simulink model "Assignment3_troubleshoot"  (R2024b)
settings: Solver=VariableStepAuto  StartTime=0.0  StopTime=0.35  MaxStep=1e-5  RelTol=1e-3
values from neighbouring files (symbols this model uses):
  C_sm = 5e-3    (= 0.005)    [assignment3.m]    (also in matlab.mat)
  Larm = 3e-3    (= 0.003)    [assignment3.m]    (also in matlab.mat)
libraries: spsIGBTDiodeLib x48, spsSeriesRLCBranchLib x30, spsVoltageMeasurementLib x28, spsTriangleGeneratorLib x24, spsCurrentMeasurementLib x9, slpidlib x5, spsabctodq0Lib x3, eeSinGeneratorThreePhase x2, spsdq0toabcLib x2, spsDCVoltageSourceLib x1, spsGroundLib x1, eePowerMeasurement x1
(part 2 of 2)

== system Assignment3_troubleshoot/Subsystem19 ==
  g : Inport
  IGBT/Diode : spsIGBTDiodeLib/IGBT//Diode  Ron=1e-3  Rs=1e5  Cs=inf  Measurements=off
  IGBT/Diode1 : spsIGBTDiodeLib/IGBT//Diode  Ron=1e-3  Rs=1e5  Cs=inf  Measurements=off
  NOT : Logic  Operator=NOT  IconShape=distinctive  AllPortsSameDT=off  OutDataTypeStr=boolean
  Series RLC Branch : spsSeriesRLCBranchLib/Series RLC Branch  LConnTagsString=__new0  RConnTagsString=__new0  BranchType=C  Resistance=1  Inductance=1e-3  SetiL0=off  InitialCurrent=0  Capacitance=C_sm  Setx0=on  InitialVoltage=V_sm  Measurements=None
  Voltage Measurement : spsVoltageMeasurementLib/Voltage Measurement  PhasorSimulation=off  OutputType=Complex  PSBequivalent=0
  1 : PMIOPort  Side=Right
  2 : PMIOPort  Port=2  Side=Right
  tag scope: Vblow_sm4=global
  wires:
  NOT/1 -> IGBT/Diode1/1
  g/1 -> IGBT/Diode/1, NOT/1
  Voltage Measurement/1 -> [Vblow_sm4]
  connections:
  IGBT/Diode/RConn1 -- 1/RConn1 -- IGBT/Diode1/LConn1
  Series RLC Branch/LConn1 -- IGBT/Diode/LConn1 -- Voltage Measurement/LConn1
  Series RLC Branch/RConn1 -- 2/RConn1 -- IGBT/Diode1/RConn1 -- Voltage Measurement/LConn2

== system Assignment3_troubleshoot/Subsystem2 ==
  g : Inport
  IGBT/Diode : spsIGBTDiodeLib/IGBT//Diode  Ron=1e-3  Rs=1e5  Cs=inf  Measurements=off
  IGBT/Diode1 : spsIGBTDiodeLib/IGBT//Diode  Ron=1e-3  Rs=1e5  Cs=inf  Measurements=off
  NOT : Logic  Operator=NOT  IconShape=distinctive  AllPortsSameDT=off  OutDataTypeStr=boolean
  Series RLC Branch : spsSeriesRLCBranchLib/Series RLC Branch  LConnTagsString=__new0  RConnTagsString=__new0  BranchType=C  Resistance=1  Inductance=1e-3  SetiL0=off  InitialCurrent=0  Capacitance=C_sm  Setx0=on  InitialVoltage=V_sm  Measurements=None
  Voltage Measurement : spsVoltageMeasurementLib/Voltage Measurement  PhasorSimulation=off  OutputType=Complex  PSBequivalent=0
  1 : PMIOPort  Side=Right
  2 : PMIOPort  Port=2  Side=Right
  tag scope: Vaup_sm3=global
  wires:
  NOT/1 -> IGBT/Diode1/1
  g/1 -> IGBT/Diode/1, NOT/1
  Voltage Measurement/1 -> [Vaup_sm3]
  connections:
  IGBT/Diode/RConn1 -- 1/RConn1 -- IGBT/Diode1/LConn1
  Series RLC Branch/LConn1 -- IGBT/Diode/LConn1 -- Voltage Measurement/LConn1
  Series RLC Branch/RConn1 -- 2/RConn1 -- IGBT/Diode1/RConn1 -- Voltage Measurement/LConn2

== system Assignment3_troubleshoot/Subsystem20 ==
  g : Inport
  IGBT/Diode : spsIGBTDiodeLib/IGBT//Diode  Ron=1e-3  Rs=1e5  Cs=inf  Measurements=off
  IGBT/Diode1 : spsIGBTDiodeLib/IGBT//Diode  Ron=1e-3  Rs=1e5  Cs=inf  Measurements=off
  NOT : Logic  Operator=NOT  IconShape=distinctive  AllPortsSameDT=off  OutDataTypeStr=boolean
  Series RLC Branch : spsSeriesRLCBranchLib/Series RLC Branch  LConnTagsString=__new0  RConnTagsString=__new0  BranchType=C  Resistance=1  Inductance=1e-3  SetiL0=off  InitialCurrent=0  Capacitance=C_sm  Setx0=on  InitialVoltage=V_sm  Measurements=None
  Voltage Measurement : spsVoltageMeasurementLib/Voltage Measurement  PhasorSimulation=off  OutputType=Complex  PSBequivalent=0
  1 : PMIOPort  Side=Right
  2 : PMIOPort  Port=2  Side=Right
  tag scope: Vclow_sm1=global
  wires:
  NOT/1 -> IGBT/Diode1/1
  g/1 -> IGBT/Diode/1, NOT/1
  Voltage Measurement/1 -> [Vclow_sm1]
  connections:
  IGBT/Diode/RConn1 -- 1/RConn1 -- IGBT/Diode1/LConn1
  Series RLC Branch/LConn1 -- IGBT/Diode/LConn1 -- Voltage Measurement/LConn1
  Series RLC Branch/RConn1 -- 2/RConn1 -- IGBT/Diode1/RConn1 -- Voltage Measurement/LConn2

== system Assignment3_troubleshoot/Subsystem21 ==
  g : Inport
  IGBT/Diode : spsIGBTDiodeLib/IGBT//Diode  Ron=1e-3  Rs=1e5  Cs=inf  Measurements=off
  IGBT/Diode1 : spsIGBTDiodeLib/IGBT//Diode  Ron=1e-3  Rs=1e5  Cs=inf  Measurements=off
  NOT : Logic  Operator=NOT  IconShape=distinctive  AllPortsSameDT=off  OutDataTypeStr=boolean
  Series RLC Branch : spsSeriesRLCBranchLib/Series RLC Branch  LConnTagsString=__new0  RConnTagsString=__new0  BranchType=C  Resistance=1  Inductance=1e-3  SetiL0=off  InitialCurrent=0  Capacitance=C_sm  Setx0=on  InitialVoltage=V_sm  Measurements=None
  Voltage Measurement : spsVoltageMeasurementLib/Voltage Measurement  PhasorSimulation=off  OutputType=Complex  PSBequivalent=0
  1 : PMIOPort  Side=Right
  2 : PMIOPort  Port=2  Side=Right
  tag scope: Vclow_sm2=global
  wires:
  NOT/1 -> IGBT/Diode1/1
  g/1 -> IGBT/Diode/1, NOT/1
  Voltage Measurement/1 -> [Vclow_sm2]
  connections:
  IGBT/Diode/RConn1 -- 1/RConn1 -- IGBT/Diode1/LConn1
  Series RLC Branch/LConn1 -- IGBT/Diode/LConn1 -- Voltage Measurement/LConn1
  Series RLC Branch/RConn1 -- 2/RConn1 -- IGBT/Diode1/RConn1 -- Voltage Measurement/LConn2

== system Assignment3_troubleshoot/Subsystem22 ==
  g : Inport
  IGBT/Diode : spsIGBTDiodeLib/IGBT//Diode  Ron=1e-3  Rs=1e5  Cs=inf  Measurements=off
  IGBT/Diode1 : spsIGBTDiodeLib/IGBT//Diode  Ron=1e-3  Rs=1e5  Cs=inf  Measurements=off
  NOT : Logic  Operator=NOT  IconShape=distinctive  AllPortsSameDT=off  OutDataTypeStr=boolean
  Series RLC Branch : spsSeriesRLCBranchLib/Series RLC Branch  LConnTagsString=__new0  RConnTagsString=__new0  BranchType=C  Resistance=1  Inductance=1e-3  SetiL0=off  InitialCurrent=0  Capacitance=C_sm  Setx0=on  InitialVoltage=V_sm  Measurements=None
  Voltage Measurement : spsVoltageMeasurementLib/Voltage Measurement  PhasorSimulation=off  OutputType=Complex  PSBequivalent=0
  1 : PMIOPort  Side=Right
  2 : PMIOPort  Port=2  Side=Right
  tag scope: Vclow_sm3=global
  wires:
  NOT/1 -> IGBT/Diode1/1
  g/1 -> IGBT/Diode/1, NOT/1
  Voltage Measurement/1 -> [Vclow_sm3]
  connections:
  IGBT/Diode/RConn1 -- 1/RConn1 -- IGBT/Diode1/LConn1
  Series RLC Branch/LConn1 -- IGBT/Diode/LConn1 -- Voltage Measurement/LConn1
  Series RLC Branch/RConn1 -- 2/RConn1 -- IGBT/Diode1/RConn1 -- Voltage Measurement/LConn2

== system Assignment3_troubleshoot/Subsystem23 ==
  g : Inport
  IGBT/Diode : spsIGBTDiodeLib/IGBT//Diode  Ron=1e-3  Rs=1e5  Cs=inf  Measurements=off
  IGBT/Diode1 : spsIGBTDiodeLib/IGBT//Diode  Ron=1e-3  Rs=1e5  Cs=inf  Measurements=off
  NOT : Logic  Operator=NOT  IconShape=distinctive  AllPortsSameDT=off  OutDataTypeStr=boolean
  Series RLC Branch : spsSeriesRLCBranchLib/Series RLC Branch  LConnTagsString=__new0  RConnTagsString=__new0  BranchType=C  Resistance=1  Inductance=1e-3  SetiL0=off  InitialCurrent=0  Capacitance=C_sm  Setx0=on  InitialVoltage=V_sm  Measurements=None
  Voltage Measurement : spsVoltageMeasurementLib/Voltage Measurement  PhasorSimulation=off  OutputType=Complex  PSBequivalent=0
  1 : PMIOPort  Side=Right
  2 : PMIOPort  Port=2  Side=Right
  tag scope: Vclow_sm4=global
  wires:
  NOT/1 -> IGBT/Diode1/1
  g/1 -> IGBT/Diode/1, NOT/1
  Voltage Measurement/1 -> [Vclow_sm4]
  connections:
  IGBT/Diode/RConn1 -- 1/RConn1 -- IGBT/Diode1/LConn1
  Series RLC Branch/LConn1 -- IGBT/Diode/LConn1 -- Voltage Measurement/LConn1
  Series RLC Branch/RConn1 -- 2/RConn1 -- IGBT/Diode1/RConn1 -- Voltage Measurement/LConn2

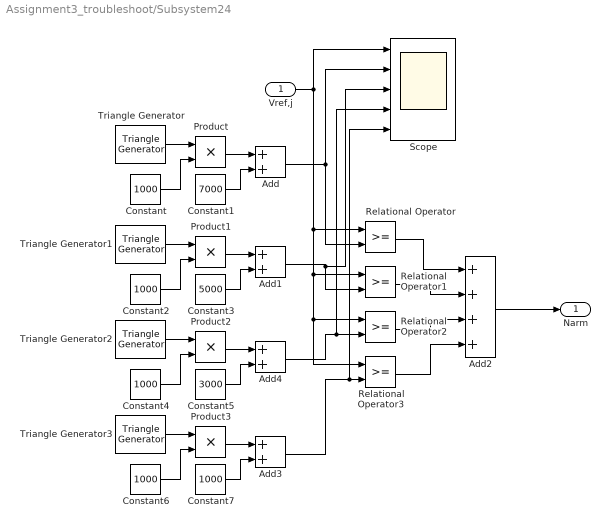
== system Assignment3_troubleshoot/Subsystem24 ==
  Vref,j : Inport
  Add{,1,3..4} (4 alike) : Sum
  Add2 : Sum  Inputs=++++
  Constant{,2,4,6..7} (5 alike) : Constant  Value=1000
  Constant1 : Constant  Value=7000
  Constant3 : Constant  Value=5000
  Constant5 : Constant  Value=3000
  Product{,1..3} (4 alike) : Product
  Relational Operator{,1..3} (4 alike) : RelationalOperator  OutDataTypeStr=boolean  RndMeth=Simplest  InputSameDT=off
  Scope : Scope  NumInputPorts=5
  Triangle Generator{,1..3} (4 alike) : spsTriangleGeneratorLib/Triangle Generator  Freq=1650  Phase=0  Ts=0
  Narm : Outport
  wires:
  Add/1 -> Relational Operator/2, Scope/2
  Product1/1 -> Add1/1
  Constant2/1 -> Product1/2
  Constant6/1 -> Product3/2
  Constant4/1 -> Product2/2
  Triangle Generator1/1 -> Product1/1
  Constant3/1 -> Add1/2
  Product3/1 -> Add3/1
  Add3/1 -> Scope/5, Relational Operator3/2
  Constant/1 -> Product/2
  Triangle Generator/1 -> Product/1
  Add1/1 -> Scope/3, Relational Operator1/2
  Add4/1 -> Scope/4, Relational Operator2/2
  Triangle Generator2/1 -> Product2/1
  Constant5/1 -> Add4/2
  Triangle Generator3/1 -> Product3/1
  Product/1 -> Add/1
  Add2/1 -> Narm/1
  Relational Operator/1 -> Add2/1
  Relational Operator3/1 -> Add2/4
  Constant1/1 -> Add/2
  Relational Operator2/1 -> Add2/3
  Vref,j/1 -> Relational Operator3/1, Relational Operator2/1, Relational Operator1/1, Relational Operator/1, Scope/1
  Constant7/1 -> Add3/2
  Relational Operator1/1 -> Add2/2
  Product2/1 -> Add4/1

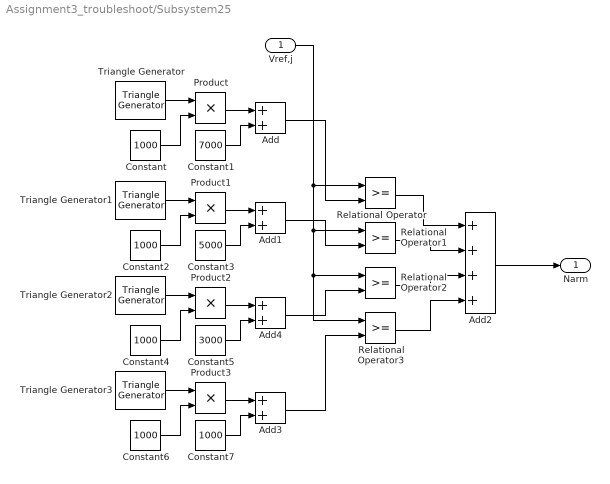
== system Assignment3_troubleshoot/Subsystem25 ==
  Vref,j : Inport
  Add{,1,3..4} (4 alike) : Sum
  Add2 : Sum  Inputs=++++
  Constant{,2,4,6..7} (5 alike) : Constant  Value=1000
  Constant1 : Constant  Value=7000
  Constant3 : Constant  Value=5000
  Constant5 : Constant  Value=3000
  Product{,1..3} (4 alike) : Product
  Relational Operator{,1..3} (4 alike) : RelationalOperator  OutDataTypeStr=boolean  RndMeth=Simplest  InputSameDT=off
  Triangle Generator{,1..3} (4 alike) : spsTriangleGeneratorLib/Triangle Generator  Freq=1650  Phase=0  Ts=0
  Narm : Outport
  wires:
  Add/1 -> Relational Operator/2
  Product1/1 -> Add1/1
  Constant2/1 -> Product1/2
  Constant6/1 -> Product3/2
  Constant4/1 -> Product2/2
  Triangle Generator1/1 -> Product1/1
  Constant3/1 -> Add1/2
  Product3/1 -> Add3/1
  Add3/1 -> Relational Operator3/2
  Constant/1 -> Product/2
  Triangle Generator/1 -> Product/1
  Add1/1 -> Relational Operator1/2
  Add4/1 -> Relational Operator2/2
  Triangle Generator2/1 -> Product2/1
  Constant5/1 -> Add4/2
  Triangle Generator3/1 -> Product3/1
  Product/1 -> Add/1
  Add2/1 -> Narm/1
  Relational Operator/1 -> Add2/1
  Relational Operator3/1 -> Add2/4
  Constant1/1 -> Add/2
  Relational Operator2/1 -> Add2/3
  Vref,j/1 -> Relational Operator3/1, Relational Operator2/1, Relational Operator1/1, Relational Operator/1
  Constant7/1 -> Add3/2
  Relational Operator1/1 -> Add2/2
  Product2/1 -> Add4/1

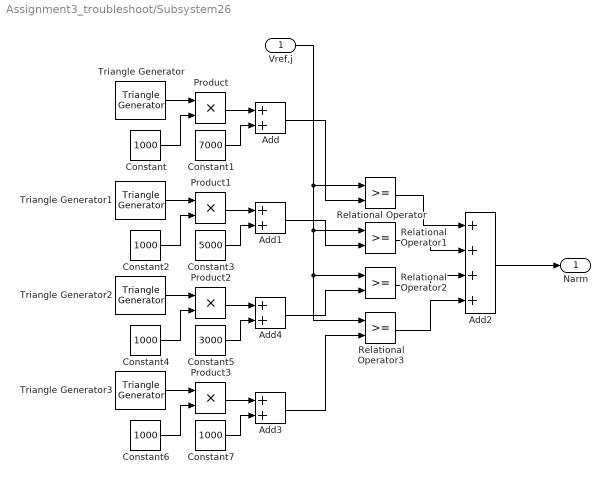
== system Assignment3_troubleshoot/Subsystem26 ==
  Vref,j : Inport
  Add{,1,3..4} (4 alike) : Sum
  Add2 : Sum  Inputs=++++
  Constant{,2,4,6..7} (5 alike) : Constant  Value=1000
  Constant1 : Constant  Value=7000
  Constant3 : Constant  Value=5000
  Constant5 : Constant  Value=3000
  Product{,1..3} (4 alike) : Product
  Relational Operator{,1..3} (4 alike) : RelationalOperator  OutDataTypeStr=boolean  RndMeth=Simplest  InputSameDT=off
  Triangle Generator{,1..3} (4 alike) : spsTriangleGeneratorLib/Triangle Generator  Freq=1650  Phase=0  Ts=0
  Narm : Outport
  wires:
  Add/1 -> Relational Operator/2
  Product1/1 -> Add1/1
  Constant2/1 -> Product1/2
  Constant6/1 -> Product3/2
  Constant4/1 -> Product2/2
  Triangle Generator1/1 -> Product1/1
  Constant3/1 -> Add1/2
  Product3/1 -> Add3/1
  Add3/1 -> Relational Operator3/2
  Constant/1 -> Product/2
  Triangle Generator/1 -> Product/1
  Add1/1 -> Relational Operator1/2
  Add4/1 -> Relational Operator2/2
  Triangle Generator2/1 -> Product2/1
  Constant5/1 -> Add4/2
  Triangle Generator3/1 -> Product3/1
  Product/1 -> Add/1
  Add2/1 -> Narm/1
  Relational Operator/1 -> Add2/1
  Relational Operator3/1 -> Add2/4
  Constant1/1 -> Add/2
  Relational Operator2/1 -> Add2/3
  Vref,j/1 -> Relational Operator3/1, Relational Operator2/1, Relational Operator1/1, Relational Operator/1
  Constant7/1 -> Add3/2
  Relational Operator1/1 -> Add2/2
  Product2/1 -> Add4/1

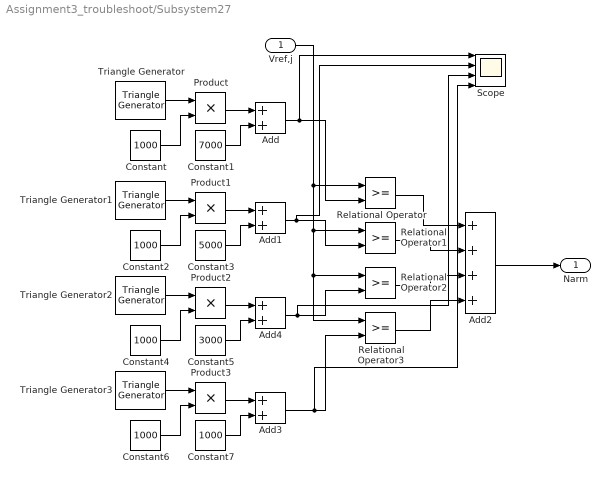
== system Assignment3_troubleshoot/Subsystem27 ==
  Vref,j : Inport
  Add{,1,3..4} (4 alike) : Sum
  Add2 : Sum  Inputs=++++
  Constant{,2,4,6..7} (5 alike) : Constant  Value=1000
  Constant1 : Constant  Value=7000
  Constant3 : Constant  Value=5000
  Constant5 : Constant  Value=3000
  Product{,1..3} (4 alike) : Product
  Relational Operator{,1..3} (4 alike) : RelationalOperator  OutDataTypeStr=boolean  RndMeth=Simplest  InputSameDT=off
  Scope : Scope  NumInputPorts=4
  Triangle Generator{,1..3} (4 alike) : spsTriangleGeneratorLib/Triangle Generator  Freq=1650  Phase=0  Ts=0
  Narm : Outport
  wires:
  Product1/1 -> Add1/1
  Constant2/1 -> Product1/2
  Constant6/1 -> Product3/2
  Constant4/1 -> Product2/2
  Triangle Generator1/1 -> Product1/1
  Constant3/1 -> Add1/2
  Product3/1 -> Add3/1
  Add3/1 -> Scope/4, Relational Operator3/2
  Constant/1 -> Product/2
  Triangle Generator/1 -> Product/1
  Add1/1 -> Scope/2, Relational Operator1/2
  Add4/1 -> Scope/3, Relational Operator2/2
  Triangle Generator2/1 -> Product2/1
  Constant5/1 -> Add4/2
  Triangle Generator3/1 -> Product3/1
  Product/1 -> Add/1
  Add2/1 -> Narm/1
  Relational Operator/1 -> Add2/1
  Relational Operator3/1 -> Add2/4
  Constant1/1 -> Add/2
  Relational Operator2/1 -> Add2/3
  Vref,j/1 -> Relational Operator3/1, Relational Operator2/1, Relational Operator1/1, Relational Operator/1
  Constant7/1 -> Add3/2
  Relational Operator1/1 -> Add2/2
  Product2/1 -> Add4/1
  Add/1 -> Scope/1, Relational Operator/2

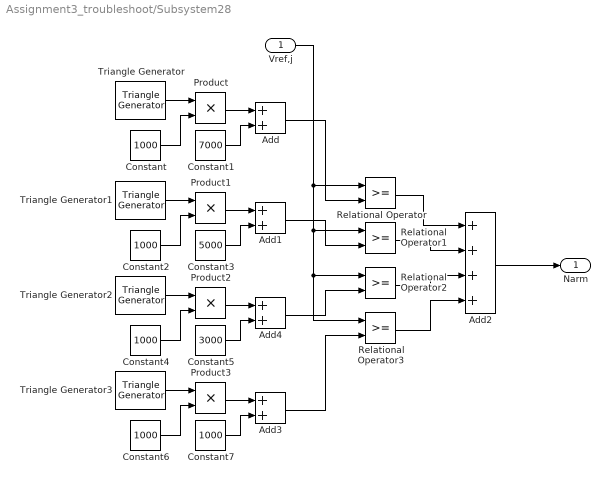
== system Assignment3_troubleshoot/Subsystem28 ==
  Vref,j : Inport
  Add{,1,3..4} (4 alike) : Sum
  Add2 : Sum  Inputs=++++
  Constant{,2,4,6..7} (5 alike) : Constant  Value=1000
  Constant1 : Constant  Value=7000
  Constant3 : Constant  Value=5000
  Constant5 : Constant  Value=3000
  Product{,1..3} (4 alike) : Product
  Relational Operator{,1..3} (4 alike) : RelationalOperator  OutDataTypeStr=boolean  RndMeth=Simplest  InputSameDT=off
  Triangle Generator{,1..3} (4 alike) : spsTriangleGeneratorLib/Triangle Generator  Freq=1650  Phase=0  Ts=0
  Narm : Outport
  wires:
  Add/1 -> Relational Operator/2
  Product1/1 -> Add1/1
  Constant2/1 -> Product1/2
  Constant6/1 -> Product3/2
  Constant4/1 -> Product2/2
  Triangle Generator1/1 -> Product1/1
  Constant3/1 -> Add1/2
  Product3/1 -> Add3/1
  Add3/1 -> Relational Operator3/2
  Constant/1 -> Product/2
  Triangle Generator/1 -> Product/1
  Add1/1 -> Relational Operator1/2
  Add4/1 -> Relational Operator2/2
  Triangle Generator2/1 -> Product2/1
  Constant5/1 -> Add4/2
  Triangle Generator3/1 -> Product3/1
  Product/1 -> Add/1
  Add2/1 -> Narm/1
  Relational Operator/1 -> Add2/1
  Relational Operator3/1 -> Add2/4
  Constant1/1 -> Add/2
  Relational Operator2/1 -> Add2/3
  Vref,j/1 -> Relational Operator3/1, Relational Operator2/1, Relational Operator1/1, Relational Operator/1
  Constant7/1 -> Add3/2
  Relational Operator1/1 -> Add2/2
  Product2/1 -> Add4/1

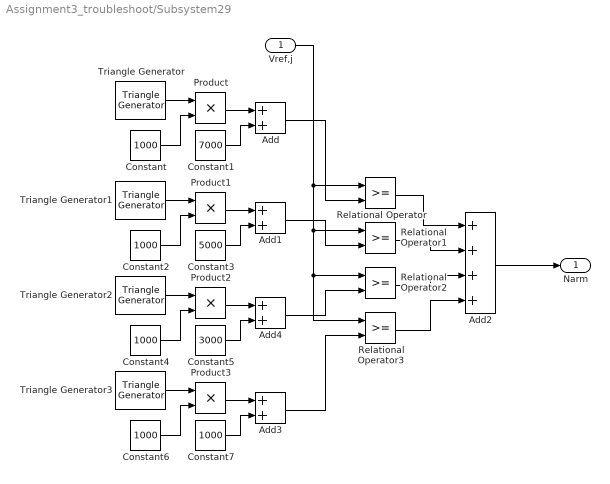
== system Assignment3_troubleshoot/Subsystem29 ==
  Vref,j : Inport
  Add{,1,3..4} (4 alike) : Sum
  Add2 : Sum  Inputs=++++
  Constant{,2,4,6..7} (5 alike) : Constant  Value=1000
  Constant1 : Constant  Value=7000
  Constant3 : Constant  Value=5000
  Constant5 : Constant  Value=3000
  Product{,1..3} (4 alike) : Product
  Relational Operator{,1..3} (4 alike) : RelationalOperator  OutDataTypeStr=boolean  RndMeth=Simplest  InputSameDT=off
  Triangle Generator{,1..3} (4 alike) : spsTriangleGeneratorLib/Triangle Generator  Freq=1650  Phase=0  Ts=0
  Narm : Outport
  wires:
  Add/1 -> Relational Operator/2
  Product1/1 -> Add1/1
  Constant2/1 -> Product1/2
  Constant6/1 -> Product3/2
  Constant4/1 -> Product2/2
  Triangle Generator1/1 -> Product1/1
  Constant3/1 -> Add1/2
  Product3/1 -> Add3/1
  Add3/1 -> Relational Operator3/2
  Constant/1 -> Product/2
  Triangle Generator/1 -> Product/1
  Add1/1 -> Relational Operator1/2
  Add4/1 -> Relational Operator2/2
  Triangle Generator2/1 -> Product2/1
  Constant5/1 -> Add4/2
  Triangle Generator3/1 -> Product3/1
  Product/1 -> Add/1
  Add2/1 -> Narm/1
  Relational Operator/1 -> Add2/1
  Relational Operator3/1 -> Add2/4
  Constant1/1 -> Add/2
  Relational Operator2/1 -> Add2/3
  Vref,j/1 -> Relational Operator3/1, Relational Operator2/1, Relational Operator1/1, Relational Operator/1
  Constant7/1 -> Add3/2
  Relational Operator1/1 -> Add2/2
  Product2/1 -> Add4/1

== system Assignment3_troubleshoot/Subsystem3 ==
  g : Inport
  IGBT/Diode : spsIGBTDiodeLib/IGBT//Diode  Ron=1e-3  Rs=1e5  Cs=inf  Measurements=off
  IGBT/Diode1 : spsIGBTDiodeLib/IGBT//Diode  Ron=1e-3  Rs=1e5  Cs=inf  Measurements=off
  NOT : Logic  Operator=NOT  IconShape=distinctive  AllPortsSameDT=off  OutDataTypeStr=boolean
  Series RLC Branch : spsSeriesRLCBranchLib/Series RLC Branch  LConnTagsString=__new0  RConnTagsString=__new0  BranchType=C  Resistance=1  Inductance=1e-3  SetiL0=off  InitialCurrent=0  Capacitance=C_sm  Setx0=on  InitialVoltage=V_sm  Measurements=None
  Voltage Measurement : spsVoltageMeasurementLib/Voltage Measurement  PhasorSimulation=off  OutputType=Complex  PSBequivalent=0
  1 : PMIOPort  Side=Right
  2 : PMIOPort  Port=2  Side=Right
  tag scope: Vaup_sm4=global
  wires:
  NOT/1 -> IGBT/Diode1/1
  g/1 -> IGBT/Diode/1, NOT/1
  Voltage Measurement/1 -> [Vaup_sm4]
  connections:
  IGBT/Diode/RConn1 -- 1/RConn1 -- IGBT/Diode1/LConn1
  Series RLC Branch/LConn1 -- IGBT/Diode/LConn1 -- Voltage Measurement/LConn1
  Series RLC Branch/RConn1 -- 2/RConn1 -- IGBT/Diode1/RConn1 -- Voltage Measurement/LConn2

== system Assignment3_troubleshoot/Subsystem4 ==
  g : Inport
  IGBT/Diode : spsIGBTDiodeLib/IGBT//Diode  Ron=1e-3  Rs=1e5  Cs=inf  Measurements=off
  IGBT/Diode1 : spsIGBTDiodeLib/IGBT//Diode  Ron=1e-3  Rs=1e5  Cs=inf  Measurements=off
  NOT : Logic  Operator=NOT  IconShape=distinctive  AllPortsSameDT=off  OutDataTypeStr=boolean
  Series RLC Branch : spsSeriesRLCBranchLib/Series RLC Branch  LConnTagsString=__new0  RConnTagsString=__new0  BranchType=C  Resistance=1  Inductance=1e-3  SetiL0=off  InitialCurrent=0  Capacitance=C_sm  Setx0=on  InitialVoltage=V_sm  Measurements=None
  Voltage Measurement : spsVoltageMeasurementLib/Voltage Measurement  PhasorSimulation=off  OutputType=Complex  PSBequivalent=0
  1 : PMIOPort  Side=Right
  2 : PMIOPort  Port=2  Side=Right
  tag scope: Valow_sm1=global
  wires:
  NOT/1 -> IGBT/Diode1/1
  g/1 -> IGBT/Diode/1, NOT/1
  Voltage Measurement/1 -> [Valow_sm1]
  connections:
  IGBT/Diode/RConn1 -- 1/RConn1 -- IGBT/Diode1/LConn1
  Series RLC Branch/LConn1 -- IGBT/Diode/LConn1 -- Voltage Measurement/LConn1
  Series RLC Branch/RConn1 -- 2/RConn1 -- IGBT/Diode1/RConn1 -- Voltage Measurement/LConn2

== system Assignment3_troubleshoot/Subsystem5 ==
  g : Inport
  IGBT/Diode : spsIGBTDiodeLib/IGBT//Diode  Ron=1e-3  Rs=1e5  Cs=inf  Measurements=off
  IGBT/Diode1 : spsIGBTDiodeLib/IGBT//Diode  Ron=1e-3  Rs=1e5  Cs=inf  Measurements=off
  NOT : Logic  Operator=NOT  IconShape=distinctive  AllPortsSameDT=off  OutDataTypeStr=boolean
  Series RLC Branch : spsSeriesRLCBranchLib/Series RLC Branch  LConnTagsString=__new0  RConnTagsString=__new0  BranchType=C  Resistance=1  Inductance=1e-3  SetiL0=off  InitialCurrent=0  Capacitance=C_sm  Setx0=on  InitialVoltage=V_sm  Measurements=None
  Voltage Measurement : spsVoltageMeasurementLib/Voltage Measurement  PhasorSimulation=off  OutputType=Complex  PSBequivalent=0
  1 : PMIOPort  Side=Right
  2 : PMIOPort  Port=2  Side=Right
  tag scope: Valow_sm2=global
  wires:
  NOT/1 -> IGBT/Diode1/1
  g/1 -> IGBT/Diode/1, NOT/1
  Voltage Measurement/1 -> [Valow_sm2]
  connections:
  IGBT/Diode/RConn1 -- 1/RConn1 -- IGBT/Diode1/LConn1
  Series RLC Branch/LConn1 -- IGBT/Diode/LConn1 -- Voltage Measurement/LConn1
  Series RLC Branch/RConn1 -- 2/RConn1 -- IGBT/Diode1/RConn1 -- Voltage Measurement/LConn2

== system Assignment3_troubleshoot/Subsystem6 ==
  g : Inport
  IGBT/Diode : spsIGBTDiodeLib/IGBT//Diode  Ron=1e-3  Rs=1e5  Cs=inf  Measurements=off
  IGBT/Diode1 : spsIGBTDiodeLib/IGBT//Diode  Ron=1e-3  Rs=1e5  Cs=inf  Measurements=off
  NOT : Logic  Operator=NOT  IconShape=distinctive  AllPortsSameDT=off  OutDataTypeStr=boolean
  Series RLC Branch : spsSeriesRLCBranchLib/Series RLC Branch  LConnTagsString=__new0  RConnTagsString=__new0  BranchType=C  Resistance=1  Inductance=1e-3  SetiL0=off  InitialCurrent=0  Capacitance=C_sm  Setx0=on  InitialVoltage=V_sm  Measurements=None
  Voltage Measurement : spsVoltageMeasurementLib/Voltage Measurement  PhasorSimulation=off  OutputType=Complex  PSBequivalent=0
  1 : PMIOPort  Side=Right
  2 : PMIOPort  Port=2  Side=Right
  tag scope: Valow_sm3=global
  wires:
  NOT/1 -> IGBT/Diode1/1
  g/1 -> IGBT/Diode/1, NOT/1
  Voltage Measurement/1 -> [Valow_sm3]
  connections:
  IGBT/Diode/RConn1 -- 1/RConn1 -- IGBT/Diode1/LConn1
  Series RLC Branch/LConn1 -- IGBT/Diode/LConn1 -- Voltage Measurement/LConn1
  Series RLC Branch/RConn1 -- 2/RConn1 -- IGBT/Diode1/RConn1 -- Voltage Measurement/LConn2

== system Assignment3_troubleshoot/Subsystem7 ==
  g : Inport
  IGBT/Diode : spsIGBTDiodeLib/IGBT//Diode  Ron=1e-3  Rs=1e5  Cs=inf  Measurements=off
  IGBT/Diode1 : spsIGBTDiodeLib/IGBT//Diode  Ron=1e-3  Rs=1e5  Cs=inf  Measurements=off
  NOT : Logic  Operator=NOT  IconShape=distinctive  AllPortsSameDT=off  OutDataTypeStr=boolean
  Series RLC Branch : spsSeriesRLCBranchLib/Series RLC Branch  LConnTagsString=__new0  RConnTagsString=__new0  BranchType=C  Resistance=1  Inductance=1e-3  SetiL0=off  InitialCurrent=0  Capacitance=C_sm  Setx0=on  InitialVoltage=V_sm  Measurements=None
  Voltage Measurement : spsVoltageMeasurementLib/Voltage Measurement  PhasorSimulation=off  OutputType=Complex  PSBequivalent=0
  1 : PMIOPort  Side=Right
  2 : PMIOPort  Port=2  Side=Right
  tag scope: Valow_sm4=global
  wires:
  NOT/1 -> IGBT/Diode1/1
  g/1 -> IGBT/Diode/1, NOT/1
  Voltage Measurement/1 -> [Valow_sm4]
  connections:
  IGBT/Diode/RConn1 -- 1/RConn1 -- IGBT/Diode1/LConn1
  Series RLC Branch/LConn1 -- IGBT/Diode/LConn1 -- Voltage Measurement/LConn1
  Series RLC Branch/RConn1 -- 2/RConn1 -- IGBT/Diode1/RConn1 -- Voltage Measurement/LConn2

== system Assignment3_troubleshoot/Subsystem8 ==
  g : Inport
  IGBT/Diode : spsIGBTDiodeLib/IGBT//Diode  Ron=1e-3  Rs=1e5  Cs=inf  Measurements=off
  IGBT/Diode1 : spsIGBTDiodeLib/IGBT//Diode  Ron=1e-3  Rs=1e5  Cs=inf  Measurements=off
  NOT : Logic  Operator=NOT  IconShape=distinctive  AllPortsSameDT=off  OutDataTypeStr=boolean
  Series RLC Branch : spsSeriesRLCBranchLib/Series RLC Branch  LConnTagsString=__new0  RConnTagsString=__new0  BranchType=C  Resistance=1  Inductance=1e-3  SetiL0=off  InitialCurrent=0  Capacitance=C_sm  Setx0=on  InitialVoltage=V_sm  Measurements=None
  Voltage Measurement : spsVoltageMeasurementLib/Voltage Measurement  PhasorSimulation=off  OutputType=Complex  PSBequivalent=0
  1 : PMIOPort  Side=Right
  2 : PMIOPort  Port=2  Side=Right
  tag scope: Vbup_sm1=global
  wires:
  NOT/1 -> IGBT/Diode1/1
  g/1 -> IGBT/Diode/1, NOT/1
  Voltage Measurement/1 -> [Vbup_sm1]
  connections:
  IGBT/Diode/RConn1 -- 1/RConn1 -- IGBT/Diode1/LConn1
  Series RLC Branch/LConn1 -- IGBT/Diode/LConn1 -- Voltage Measurement/LConn1
  Series RLC Branch/RConn1 -- 2/RConn1 -- IGBT/Diode1/RConn1 -- Voltage Measurement/LConn2

== system Assignment3_troubleshoot/Subsystem9 ==
  g : Inport
  IGBT/Diode : spsIGBTDiodeLib/IGBT//Diode  Ron=1e-3  Rs=1e5  Cs=inf  Measurements=off
  IGBT/Diode1 : spsIGBTDiodeLib/IGBT//Diode  Ron=1e-3  Rs=1e5  Cs=inf  Measurements=off
  NOT : Logic  Operator=NOT  IconShape=distinctive  AllPortsSameDT=off  OutDataTypeStr=boolean
  Series RLC Branch : spsSeriesRLCBranchLib/Series RLC Branch  LConnTagsString=__new0  RConnTagsString=__new0  BranchType=C  Resistance=1  Inductance=1e-3  SetiL0=off  InitialCurrent=0  Capacitance=C_sm  Setx0=on  InitialVoltage=V_sm  Measurements=None
  Voltage Measurement : spsVoltageMeasurementLib/Voltage Measurement  PhasorSimulation=off  OutputType=Complex  PSBequivalent=0
  1 : PMIOPort  Side=Right
  2 : PMIOPort  Port=2  Side=Right
  tag scope: Vbup_sm2=global
  wires:
  NOT/1 -> IGBT/Diode1/1
  g/1 -> IGBT/Diode/1, NOT/1
  Voltage Measurement/1 -> [Vbup_sm2]
  connections:
  IGBT/Diode/RConn1 -- 1/RConn1 -- IGBT/Diode1/LConn1
  Series RLC Branch/LConn1 -- IGBT/Diode/LConn1 -- Voltage Measurement/LConn1
  Series RLC Branch/RConn1 -- 2/RConn1 -- IGBT/Diode1/RConn1 -- Voltage Measurement/LConn2

== matlab function Assignment3_troubleshoot/MATLAB Function ==
  data: V_C1 input; V_C2 input; V_C3 input; V_C4 input; i_arm input; N_insert input; S1 output; S2 output; S3 output; S4 output
function [S1, S2, S3, S4] = voltage_balancing(V_C1, V_C2, V_C3, V_C4, i_arm, N_insert)
    
    % Create array: [SM_index, voltage]
    SM_array = [1, V_C1;
                2, V_C2;
                3, V_C3;
                4, V_C4];
    
    % Sort based on current direction
    if i_arm > 0
        % Charging: sort ascending (lowest voltage first)
        [~, sort_idx] = sort(SM_array(:,2), 'ascend');
    else
        % Discharging: sort descending (highest voltage first)
        [~, sort_idx] = sort(SM_array(:,2), 'descend');
    end
    
    % Reorder based on sorted indices
    SM_sorted = SM_array(sort_idx, :);
    
    % Select first N_insert SMs
    selected_indices = SM_sorted(1:N_insert, 1);
    
    % Generate gate signals (1 if selected, 0 if not)
    S1 = any(selected_indices == 1);
    S2 = any(selected_indices == 2);
    S3 = any(selected_indices == 3);
    S4 = any(selected_indices == 4);
    
end

== matlab function Assignment3_troubleshoot/MATLAB Function1 ==
  data: V_C1 input; V_C2 input; V_C3 input; V_C4 input; i_arm input; N_insert input; S1 output; S2 output; S3 output; S4 output
function [S1, S2, S3, S4] = voltage_balancing(V_C1, V_C2, V_C3, V_C4, i_arm, N_insert)
    
    % Create array: [SM_index, voltage]
    SM_array = [1, V_C1;
                2, V_C2;
                3, V_C3;
                4, V_C4];
    
    % Sort based on current direction
    if i_arm > 0
        % Charging: sort ascending (lowest voltage first)
        [~, sort_idx] = sort(SM_array(:,2), 'ascend');
    else
        % Discharging: sort descending (highest voltage first)
        [~, sort_idx] = sort(SM_array(:,2), 'descend');
    end
    
    % Reorder based on sorted indices
    SM_sorted = SM_array(sort_idx, :);
    
    % Select first N_insert SMs
    selected_indices = SM_sorted(1:N_insert, 1);
    
    % Generate gate signals (1 if selected, 0 if not)
    S1 = any(selected_indices == 1);
    S2 = any(selected_indices == 2);
    S3 = any(selected_indices == 3);
    S4 = any(selected_indices == 4);
    
end

== matlab function Assignment3_troubleshoot/MATLAB Function2 ==
  data: V_C1 input; V_C2 input; V_C3 input; V_C4 input; i_arm input; N_insert input; S1 output; S2 output; S3 output; S4 output
function [S1, S2, S3, S4] = voltage_balancing(V_C1, V_C2, V_C3, V_C4, i_arm, N_insert)
    
    % Create array: [SM_index, voltage]
    SM_array = [1, V_C1;
                2, V_C2;
                3, V_C3;
                4, V_C4];
    
    % Sort based on current direction
    if i_arm > 0
        % Charging: sort ascending (lowest voltage first)
        [~, sort_idx] = sort(SM_array(:,2), 'ascend');
    else
        % Discharging: sort descending (highest voltage first)
        [~, sort_idx] = sort(SM_array(:,2), 'descend');
    end
    
    % Reorder based on sorted indices
    SM_sorted = SM_array(sort_idx, :);
    
    % Select first N_insert SMs
    selected_indices = SM_sorted(1:N_insert, 1);
    
    % Generate gate signals (1 if selected, 0 if not)
    S1 = any(selected_indices == 1);
    S2 = any(selected_indices == 2);
    S3 = any(selected_indices == 3);
    S4 = any(selected_indices == 4);
    
end

== matlab function Assignment3_troubleshoot/MATLAB Function3 ==
  data: V_C1 input; V_C2 input; V_C3 input; V_C4 input; i_arm input; N_insert input; S1 output; S2 output; S3 output; S4 output
function [S1, S2, S3, S4] = voltage_balancing(V_C1, V_C2, V_C3, V_C4, i_arm, N_insert)
    
    % Create array: [SM_index, voltage]
    SM_array = [1, V_C1;
                2, V_C2;
                3, V_C3;
                4, V_C4];
    
    % Sort based on current direction
    if i_arm > 0
        % Charging: sort ascending (lowest voltage first)
        [~, sort_idx] = sort(SM_array(:,2), 'ascend');
    else
        % Discharging: sort descending (highest voltage first)
        [~, sort_idx] = sort(SM_array(:,2), 'descend');
    end
    
    % Reorder based on sorted indices
    SM_sorted = SM_array(sort_idx, :);
    
    % Select first N_insert SMs
    selected_indices = SM_sorted(1:N_insert, 1);
    
    % Generate gate signals (1 if selected, 0 if not)
    S1 = any(selected_indices == 1);
    S2 = any(selected_indices == 2);
    S3 = any(selected_indices == 3);
    S4 = any(selected_indices == 4);
    
end

== matlab function Assignment3_troubleshoot/MATLAB Function4 ==
  data: V_C1 input; V_C2 input; V_C3 input; V_C4 input; i_arm input; N_insert input; S1 output; S2 output; S3 output; S4 output
function [S1, S2, S3, S4] = voltage_balancing(V_C1, V_C2, V_C3, V_C4, i_arm, N_insert)
    
    % Create array: [SM_index, voltage]
    SM_array = [1, V_C1;
                2, V_C2;
                3, V_C3;
                4, V_C4];
    
    % Sort based on current direction
    if i_arm > 0
        % Charging: sort ascending (lowest voltage first)
        [~, sort_idx] = sort(SM_array(:,2), 'ascend');
    else
        % Discharging: sort descending (highest voltage first)
        [~, sort_idx] = sort(SM_array(:,2), 'descend');
    end
    
    % Reorder based on sorted indices
    SM_sorted = SM_array(sort_idx, :);
    
    % Select first N_insert SMs
    selected_indices = SM_sorted(1:N_insert, 1);
    
    % Generate gate signals (1 if selected, 0 if not)
    S1 = any(selected_indices == 1);
    S2 = any(selected_indices == 2);
    S3 = any(selected_indices == 3);
    S4 = any(selected_indices == 4);
    
end

== matlab function Assignment3_troubleshoot/MATLAB Function5 ==
  data: V_C1 input; V_C2 input; V_C3 input; V_C4 input; i_arm input; N_insert input; S1 output; S2 output; S3 output; S4 output
function [S1, S2, S3, S4] = voltage_balancing(V_C1, V_C2, V_C3, V_C4, i_arm, N_insert)
    
    % Create array: [SM_index, voltage]
    SM_array = [1, V_C1;
                2, V_C2;
                3, V_C3;
                4, V_C4];
    
    % Sort based on current direction
    if i_arm > 0
        % Charging: sort ascending (lowest voltage first)
        [~, sort_idx] = sort(SM_array(:,2), 'ascend');
    else
        % Discharging: sort descending (highest voltage first)
        [~, sort_idx] = sort(SM_array(:,2), 'descend');
    end
    
    % Reorder based on sorted indices
    SM_sorted = SM_array(sort_idx, :);
    
    % Select first N_insert SMs
    selected_indices = SM_sorted(1:N_insert, 1);
    
    % Generate gate signals (1 if selected, 0 if not)
    S1 = any(selected_indices == 1);
    S2 = any(selected_indices == 2);
    S3 = any(selected_indices == 3);
    S4 = any(selected_indices == 4);
    
end
